simulink model "stp1_8sym"  (R2022b)
settings: Solver=VariableStepAuto  StartTime=0.0  StopTime=35  RelTol=1e-3
values from neighbouring files (symbols this model uses):
  B_gain = 1.5    [stp1.m]
  K2 = Kr(1:3)    [stp1.m]
  Ke = Kr(4)    [stp1.m]
settings Model: Creator=zalew  LastModifiedBy=zalew

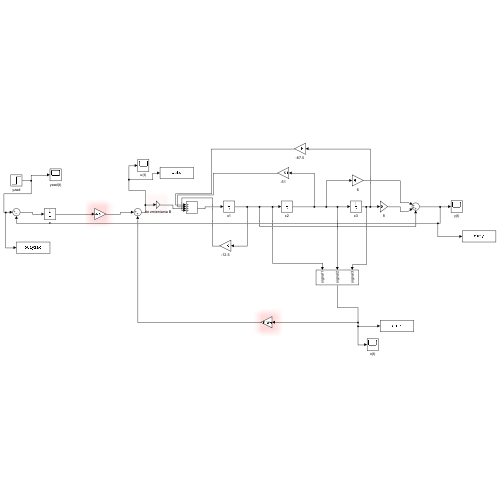
[thumbnail: Simulink's stored preview of the top-level diagram]
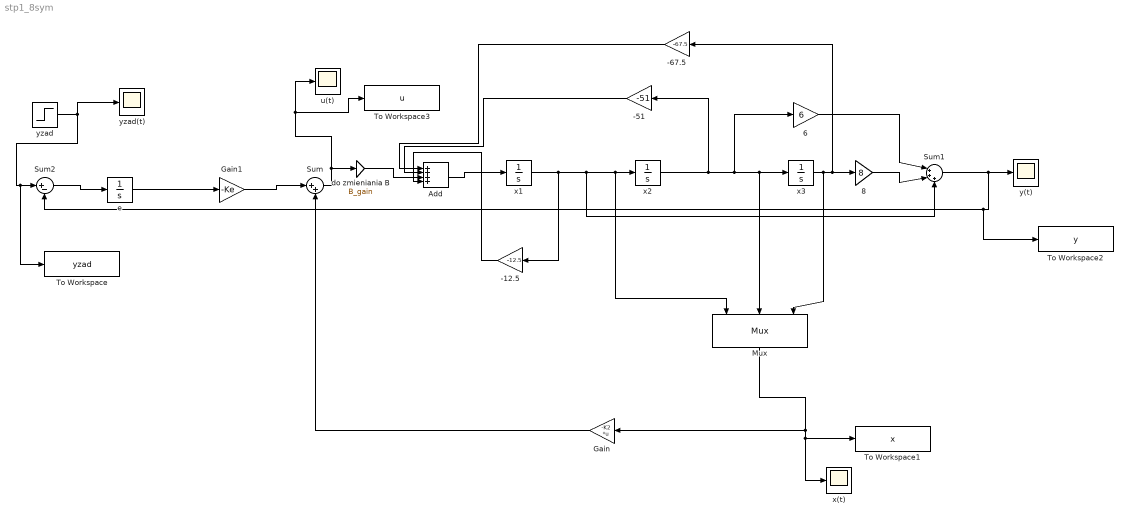
== system stp1_8sym ==
  -12.5 : Gain  Gain=-12.5
  -51 : Gain  Gain=-51
  -67.5 : Gain  Gain=-67.5
  6 : Gain  Gain=6
  8 : Gain  Gain=8
  Add : Sum  Inputs=++++
  Gain : Gain  Gain=-K2  Multiplication=Matrix(K*u) (u vector)
  Gain1 : Gain  Gain=-Ke
  Mux : Mux  Inputs=3
      settings: DisplayOption=signals
  Sum : Sum  Inputs=|++
  Sum1 : Sum  Inputs=|+++
  Sum2 : Sum  Inputs=|+-
  To Workspace : ToWorkspace  VariableName=yzad  SaveFormat=Timeseries  SampleTime=-1
  To Workspace1 : ToWorkspace  VariableName=x  SaveFormat=Timeseries  SampleTime=-1
  To Workspace2 : ToWorkspace  VariableName=y  SaveFormat=Timeseries  SampleTime=-1
  To Workspace3 : ToWorkspace  VariableName=u  SaveFormat=Timeseries  SampleTime=-1
  do zmieniania B : Gain  Gain=B_gain
  e : Integrator
  u(t) : Scope
  x(t) : Scope
  x1 : Integrator
  x2 : Integrator
  x3 : Integrator
  y(t) : Scope
  yzad : Step  Time=10  After=5  SampleTime=0
  yzad(t) : Scope
  wires:
  x3/1 -> Mux/3, -67.5/1, 8/1
  -12.5/1 -> Add/4
  Sum1/1 -> To Workspace2/1, Sum2/2, y(t)/1
  6/1 -> Sum1/1
  x2/1 -> x3/1, Mux/2, 6/1, -51/1
  -67.5/1 -> Add/1
  8/1 -> Sum1/2
  Add/1 -> x1/1
  -51/1 -> Add/2
  x1/1 -> -12.5/1, Mux/1, x2/1, Sum1/3
  Mux/1 -> x(t)/1, To Workspace1/1, Gain/1
  Gain/1 -> Sum/2
  Sum/1 -> do zmieniania B/1, To Workspace3/1, u(t)/1
  Gain1/1 -> Sum/1
  Sum2/1 -> e/1
  yzad/1 -> To Workspace/1, Sum2/1, yzad(t)/1
  e/1 -> Gain1/1
  do zmieniania B/1 -> Add/3
